simulink model "diodeModel"  (R2020a)
settings: Solver=VariableStepAuto  StartTime=0.0  StopTime=10  RelTol=1e-3
values from neighbouring files (symbols this model uses):
  current = union(in,ip)    [lookupTableScript.m]
  voltage = [-51:0.1:1]    [lookupTableScript.m]
settings Model: Creator=DELL  LastModifiedBy=DELL
settings DataIOCC: ExternalInput=[t,voltage]

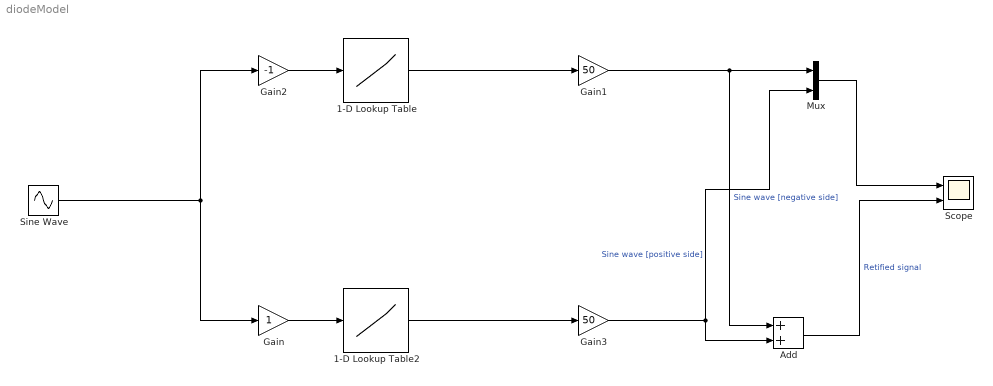
== system diodeModel ==
  1-D Lookup Table : Lookup_n-D  NumberOfTableDimensions=1  BreakpointsForDimension1=voltage  Table=current  InternalRulePriority=Speed  RndMeth=Simplest  InputSameDT=on
  1-D Lookup Table2 : Lookup_n-D  NumberOfTableDimensions=1  BreakpointsForDimension1=voltage  Table=current  InternalRulePriority=Speed  RndMeth=Simplest  InputSameDT=on
  Add : Sum
  Gain : Gain
  Gain1 : Gain  Gain=50
  Gain2 : Gain  Gain=-1
  Gain3 : Gain  Gain=50
  Mux : Mux  Inputs=2
  Scope : Scope  NumInputPorts=2
  Sine Wave : Sin  Amplitude=2  SampleTime=0
  wires:
  1-D Lookup Table/1 -> Gain1/1
  Gain1/1 -> Add/1, Mux/1  "Sine wave [negative side]"
  Gain3/1 -> Add/2, Mux/2  "Sine wave [positive side]"
  1-D Lookup Table2/1 -> Gain3/1
  Sine Wave/1 -> Gain/1, Gain2/1
  Mux/1 -> Scope/1
  Gain2/1 -> 1-D Lookup Table/1
  Gain/1 -> 1-D Lookup Table2/1
  Add/1 -> Scope/2  "Retified signal"
